simulink model "gm_uz_pmsm_model_6ph_dqxy_vnl"  (R2024b)
settings: Solver=FixedStepAuto  StartTime=0.0  StopTime=0.5  RelTol=1e-3
PreLoadFcn:
  | uz_pmsm_model_6ph_dqxy_init_parameter
undefined symbols (not defined in the file or in its folder): friction_coefficient, inertia, k_i_d, k_i_x, k_i_y, k_p_d, k_p_q, k_p_x, k_p_y, L_d, L_q, L_x, L_y, polepair, psi_pm, R_1, setpoint_step, simulate_mechanical, simulate_open_loop, static_friction_torque, ts
libraries: hdlmdlgenlib x5, slpidlib x4, simulink x2
(part 1 of 2)
settings Model: Creator=ts  LastModifiedBy=hufnagelde
settings SolverCC: AlgebraicLoopSolver=TrustRegion  AutoInsertRateTranBlk=on
settings DataIOCC: LimitDataPoints=on  SaveOutput=off  SaveTime=off
settings OptimizationCC: BlockReduction=off  ConditionallyExecuteInputs=off  DefaultParameterBehavior=Inlined  LifeSpan=inf
settings DebuggingCC: AlgebraicLoopMsg=error  InheritedTsInSrcMsg=none  SingleTaskRateTransMsg=error  UnconnectedInputMsg=warning  UnconnectedOutputMsg=warning  UnconnectedLineMsg=warning  AllowSymbolicDim=off  StrictBusMsg=ErrorOnBusTreatedAsVector  SFUnexpectedBacktrackingDiag=warning  SFNoUnconditionalDefaultTransitionDiag=warning  SFExecutionAtInitializationDiag=none  ArithmeticOperatorsInVariantConditions=warning
settings HardwareCC: ProdBitPerPointer=32  ProdBitPerSizeT=32  ProdBitPerPtrDiffT=32  ProdLargestAtomicFloat=None  ProdIntDivRoundTo=Undefined  ProdEndianess=Unspecified  ProdWordSize=32  ProdHWDeviceType=ASIC/FPGA->ASIC/FPGA  ProdEqTarget=off
settings ModelReferenceCC: EnableRefExpFcnMdlSchedulingChecks=on
settings SFSimCC: SimUseLocalCustomCode=off  CustomCodeUndefinedFunction=UseInterfaceOnly
settings RTWCC: RTWUseLocalCustomCode=off  GPUComputeCapability=3.5  DLArmComputeVersion=19.05
settings CodeAppCC: StateflowObjectComments=on
settings GRTTargetCC: TargetLangStandard=C89/C90 (ANSI)
settings ConfigComp: CovScope=ReferencedModels  CovMetricSettings=dw  CovSaveCumulativeToWorkspaceVar=on  CovSaveSingleToWorkspaceVar=on  CovExternalEMLEnable=off  CovSFcnEnable=off

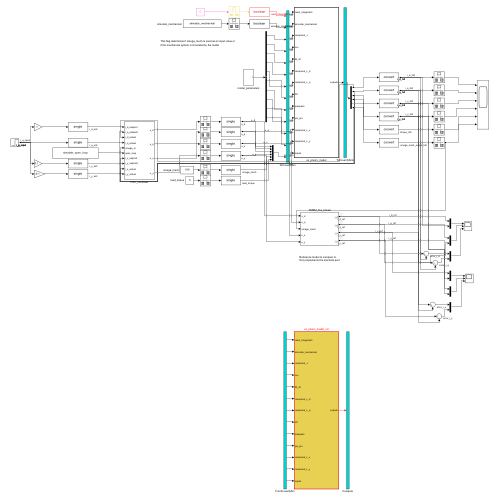
[thumbnail: Simulink's stored preview of the top-level diagram]
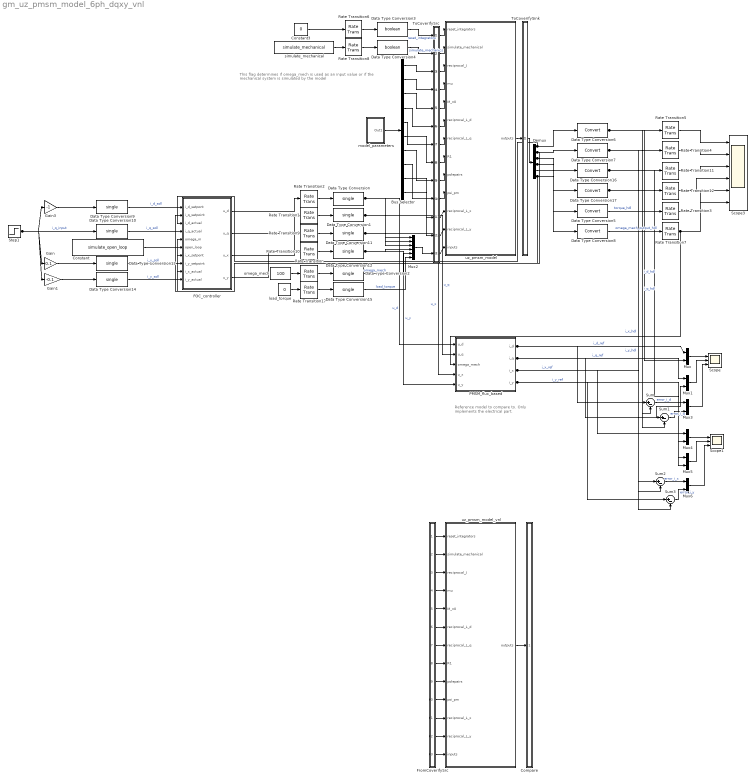
== system gm_uz_pmsm_model_6ph_dqxy_vnl ==
  note: Reference model to compare to.
      | Only implements the electrical part.
  note: This flag determines if omega_mech is used as an input value or
      | if the mechanical system is simulated by the model
  Bus Selector : BusSelector  OutputSignals=1_J,mu,M_R0,1_L_d,1_L_q,R_1,polepair,psi_pm,1_L_x,1_L_y
  Compare : Subsystem
      mask Display: disp('')
  Constant : Constant  Value=simulate_open_loop
  Constant3 : Constant  Value=0
  Data Type Conversion{,1..2,9..15} (10 alike) : DataTypeConversion  OutDataTypeStr=single  SaturateOnIntegerOverflow=off  RndMeth=Floor
  Data Type Conversion{5..8,16..17} (6 alike) : DataTypeConversion  SaturateOnIntegerOverflow=off  RndMeth=Floor
  Data Type Conversion3 : DataTypeConversion  OutDataTypeStr=boolean  SaturateOnIntegerOverflow=off  RndMeth=Floor
  Data Type Conversion4 : DataTypeConversion  OutDataTypeStr=boolean  SaturateOnIntegerOverflow=off  RndMeth=Floor
  Demux : Demux  Outputs=6
  FOC_controller : Subsystem
  FromCoverifySrc : Subsystem
      mask Display: disp('')
  Gain : Gain  Gain=0.1
  Gain1 : Gain  Gain=-0.1
  Gain3 : Gain  Gain=-1
  Mux{,1,3..6} (6 alike) : Mux  Inputs=2
  Mux2 : Mux  Inputs=6
  PMSM_flux_based : Subsystem
  Rate Transition{,1..2,6,8..10,17} (8 alike) : RateTransition  OutPortSampleTime=ts
  Rate Transition{3..5,7,11..12} (6 alike) : RateTransition
  Scope : Scope  NumInputPorts=3
  Scope1 : Scope  NumInputPorts=3
  Scope3 : Scope  NumInputPorts=6
  Step1 : Step  Time=0.2  After=setpoint_step
  Sum{,1..3} (4 alike) : Sum  Inputs=|+-
  ToCoverifySink : Subsystem
      mask Display: disp('')
  ToCoverifySrc : Subsystem
      mask Display: disp('')
  load_torque : Constant  Value=0
  model_parameters : Subsystem
  omega_mech : Constant  Value=100
  simulate_mechanical : Constant  Value=simulate_mechanical
  uz_pmsm_model : Subsystem  TreatAsAtomicUnit=on
  uz_pmsm_model_vnl : Subsystem  TreatAsAtomicUnit=on
  wires:
  Rate Transition/1 -> Data Type Conversion2/1
  Data Type Conversion6/1 -> Mux/2, Sum/2, Rate Transition5/1  "i_d_hdl"
  Data Type Conversion7/1 -> Mux1/2, Sum1/2, Rate Transition4/1  "i_q_hdl"
  Data Type Conversion5/1 -> Rate Transition3/1  "torque_hdl"
  Rate Transition4/1 -> Scope3/2
  Rate Transition5/1 -> Scope3/1
  Rate Transition3/1 -> Scope3/5
  Rate Transition6/1 -> Data Type Conversion3/1
  Constant3/1 -> Rate Transition6/1
  Rate Transition8/1 -> Data Type Conversion4/1
  simulate_mechanical/1 -> Rate Transition8/1
  load_torque/1 -> Rate Transition17/1
  Rate Transition17/1 -> Data Type Conversion15/1
  Mux/1 -> Scope/1
  Mux1/1 -> Scope/2
  PMSM_flux_based/2(i_q) -> Mux1/1, Sum1/1  "i_q_ref"
  PMSM_flux_based/1(i_d) -> Mux/1, Sum/1  "i_d_ref"
  Data Type Conversion8/1 -> Rate Transition7/1  "omega_mech_output_hdl"
  Rate Transition7/1 -> PMSM_flux_based/3(omega_mech), Scope3/6
  model_parameters/1(Out1) -> Bus Selector/1
  Sum/1 -> Mux3/1  "error_i_d"
  Sum1/1 -> Mux3/2  "error_i_q"
  Mux3/1 -> Scope/3
  Step1/1 -> Gain1/1, Gain/1, Gain3/1, Data Type Conversion10/1  "i_q_input"
  Demux/5 -> Data Type Conversion5/1
  Gain3/1 -> Data Type Conversion9/1
  Demux/1 -> FOC_controller/3(i_d_actual), Data Type Conversion6/1
  Demux/6 -> FOC_controller/5(omega_m), Data Type Conversion8/1
  Demux/2 -> FOC_controller/4(i_q_actual), Data Type Conversion7/1
  Data Type Conversion/1 -> PMSM_flux_based/1(u_d), Mux2/1  "u_d"
  Data Type Conversion1/1 -> PMSM_flux_based/2(u_q), Mux2/2  "u_q"
  Data Type Conversion15/1 -> Mux2/6  "load_torque"
  Data Type Conversion2/1 -> Mux2/5  "omega_mech"
  Data Type Conversion9/1 -> FOC_controller/1(i_d_setpont)  "i_d_soll"
  Data Type Conversion10/1 -> FOC_controller/2(i_q_setpoint)  "i_q_soll"
  omega_mech/1 -> Rate Transition/1
  Constant/1 -> FOC_controller/6(open_loop)
  Rate Transition9/1 -> Data Type Conversion11/1
  Rate Transition10/1 -> Data Type Conversion12/1
  Rate Transition1/1 -> Data Type Conversion1/1
  Rate Transition2/1 -> Data Type Conversion/1
  FOC_controller/1(u_d) -> Rate Transition2/1
  FOC_controller/2(u_q) -> Rate Transition1/1
  FOC_controller/3(u_x) -> Rate Transition9/1
  FOC_controller/4(u_y) -> Rate Transition10/1
  Data Type Conversion11/1 -> PMSM_flux_based/4(u_x), Mux2/3  "u_x"
  Data Type Conversion12/1 -> PMSM_flux_based/5(u_y), Mux2/4  "u_y"
  Gain1/1 -> Data Type Conversion14/1
  Gain/1 -> Data Type Conversion13/1
  Data Type Conversion13/1 -> FOC_controller/7(i_x_setpont)  "i_x_soll"
  Data Type Conversion14/1 -> FOC_controller/8(i_y_setpoint)  "i_y_soll"
  Data Type Conversion16/1 -> Sum2/2, Mux4/2, Rate Transition11/1  "i_x_hdl"
  Rate Transition11/1 -> Scope3/3
  Demux/3 -> FOC_controller/9(i_x_actual), Data Type Conversion16/1
  Data Type Conversion17/1 -> Sum3/2, Mux5/2, Rate Transition12/1  "i_y_hdl"
  Rate Transition12/1 -> Scope3/4
  Demux/4 -> FOC_controller/10(i_y_actual), Data Type Conversion17/1
  Mux4/1 -> Scope1/1
  PMSM_flux_based/3(i_x) -> Sum2/1, Mux4/1  "i_x_ref"
  PMSM_flux_based/4(i_y) -> Mux5/1, Sum3/1  "i_y_ref"
  Mux5/1 -> Scope1/2
  Sum2/1 -> Mux6/1  "error_i_x"
  Sum3/1 -> Mux6/2  "error_i_y"
  Mux6/1 -> Scope1/3
  ToCoverifySrc/1(out1) -> uz_pmsm_model/1(reset_integrators)
  ToCoverifySrc/2(out2) -> uz_pmsm_model/2(simulate_mechanical)
  ToCoverifySrc/3(out3) -> uz_pmsm_model/3(reciprocal_J)
  ToCoverifySrc/4(out4) -> uz_pmsm_model/4(mu)
  ToCoverifySrc/5(out5) -> uz_pmsm_model/5(M_n0)
  ToCoverifySrc/6(out6) -> uz_pmsm_model/6(reciprocal_L_d)
  ToCoverifySrc/7(out7) -> uz_pmsm_model/7(reciprocal_L_q)
  ToCoverifySrc/8(out8) -> uz_pmsm_model/8(R1)
  ToCoverifySrc/9(out9) -> uz_pmsm_model/9(polepairs)
  ToCoverifySrc/10(out10) -> uz_pmsm_model/10(psi_pm)
  ToCoverifySrc/11(out11) -> uz_pmsm_model/11(reciprocal_L_x)
  ToCoverifySrc/12(out12) -> uz_pmsm_model/12(reciprocal_L_y)
  ToCoverifySrc/13(out13) -> uz_pmsm_model/13(inputs)
  uz_pmsm_model/1(outputs) -> ToCoverifySink/1(in1)
  Data Type Conversion3/1 -> ToCoverifySrc/1(in1)  "reset_integrators"
  Data Type Conversion4/1 -> ToCoverifySrc/2(in2)  "simulate_mechanics"
  Bus Selector/1 -> ToCoverifySrc/3(in3)
  Bus Selector/2 -> ToCoverifySrc/4(in4)
  Bus Selector/3 -> ToCoverifySrc/5(in5)
  Bus Selector/4 -> ToCoverifySrc/6(in6)
  Bus Selector/5 -> ToCoverifySrc/7(in7)
  Bus Selector/6 -> ToCoverifySrc/8(in8)
  Bus Selector/7 -> ToCoverifySrc/9(in9)
  Bus Selector/8 -> ToCoverifySrc/10(in10)
  Bus Selector/9 -> ToCoverifySrc/11(in11)
  Bus Selector/10 -> ToCoverifySrc/12(in12)
  Mux2/1 -> ToCoverifySrc/13(in13)
  ToCoverifySink/1(out1) -> Demux/1
  FromCoverifySrc/1(out1) -> uz_pmsm_model_vnl/1(reset_integrators)
  FromCoverifySrc/2(out2) -> uz_pmsm_model_vnl/2(simulate_mechanical)
  FromCoverifySrc/3(out3) -> uz_pmsm_model_vnl/3(reciprocal_J)
  FromCoverifySrc/4(out4) -> uz_pmsm_model_vnl/4(mu)
  FromCoverifySrc/5(out5) -> uz_pmsm_model_vnl/5(M_n0)
  FromCoverifySrc/6(out6) -> uz_pmsm_model_vnl/6(reciprocal_L_d)
  FromCoverifySrc/7(out7) -> uz_pmsm_model_vnl/7(reciprocal_L_q)
  FromCoverifySrc/8(out8) -> uz_pmsm_model_vnl/8(R1)
  FromCoverifySrc/9(out9) -> uz_pmsm_model_vnl/9(polepairs)
  FromCoverifySrc/10(out10) -> uz_pmsm_model_vnl/10(psi_pm)
  FromCoverifySrc/11(out11) -> uz_pmsm_model_vnl/11(reciprocal_L_x)
  FromCoverifySrc/12(out12) -> uz_pmsm_model_vnl/12(reciprocal_L_y)
  FromCoverifySrc/13(out13) -> uz_pmsm_model_vnl/13(inputs)
  uz_pmsm_model_vnl/1(outputs) -> Compare/1(in1)

== system gm_uz_pmsm_model_6ph_dqxy_vnl/Compare ==
  in1 : Inport
  Assert_outputs : Subsystem  mask{ToleranceValue=1e-07}
  CleanupScopes : Subsystem
      settings: OpenFcn=|
      | blkName = gcb; %self block
      | idx = regexp(blkName, '/CleanupScopes$', 'once');
      | blkParent = blkName(1:idx-1);
      | blks=find_system(blkParent, 'LookUnderMasks', 'all','blocktype', 'Scope');
      | for itr = 1:length(blks)
      | 	 hScopeCfg = get_param(blks{itr},'ScopeConfiguration');
      | 	 hScopeCfg.Visible = ~ hScopeCfg.Visible;
      | end
      | drawnow;
      mask Display: fprintf(message('hdlcoder:cosim:vnl_dblclick').getString());
  Enable : Subsystem
      settings: OpenFcn=|
      | blkName = gcb;
      | idx = regexp(blkName, '/Enable$', 'once');
      | blkParent = blkName(1:idx-1);
      | blks=find_system(blkParent, 'LookUnderMasks', 'all','blocktype', 'Assertion');
      | e = get_param(blks{1}, 'Enabled');
      | if strcmp(e, 'on'), f= 'off';, else, f = 'on';, end
      | for ii=1:length(blks), set_param(blks{ii}, 'Enabled', f);, end
      | set_param(gcb, 'MaskDisplay',['fprintf(message(''hdlcoder:cosim:vnl_dblclick_assertions'',','''',upper(e),'''',').getString())']);
      mask Display: fprintf(message('hdlcoder:cosim:vnl_dblclick_assertions','OFF').getString());
  pathdelay1 : Delay  DelayLength=1
  wires:
  in1/1 -> pathdelay1/1
  pathdelay1/1 -> Assert_outputs/1(cosim)
  [out1] -> Assert_outputs/2(dut)

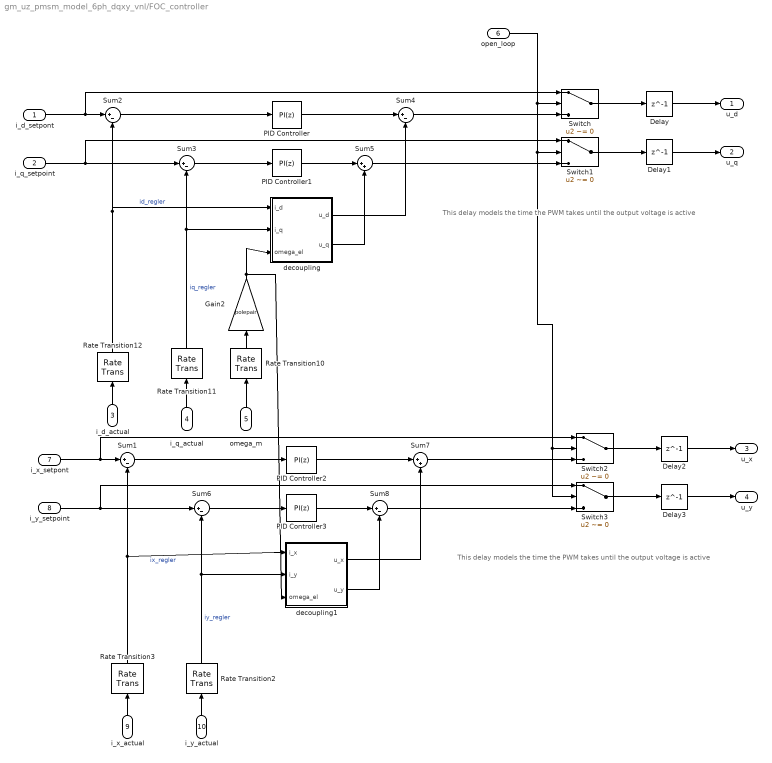
== system gm_uz_pmsm_model_6ph_dqxy_vnl/FOC_controller ==
  note: This delay models the time the PWM takes until the output voltage is active
  note: This delay models the time the PWM takes until the output voltage is active
  i_d_setpont : Inport
  i_q_setpoint : Inport  Port=2
  i_d_actual : Inport  Port=3
  i_q_actual : Inport  Port=4
  omega_m : Inport  Port=5
  open_loop : Inport  Port=6
  i_x_setpont : Inport  Port=7
  i_y_setpoint : Inport  Port=8
  i_x_actual : Inport  Port=9
  i_y_actual : Inport  Port=10
  Delay{,1..3} (4 alike) : Delay  DelayLength=1
  Gain2 : Gain  Gain=polepair
  PID Controller : slpidlib/PID Controller  Controller=PI  Form=Parallel  TimeDomain=Discrete-time  UseExternalTs=off  SampleTime=-1  IntegratorMethod=Forward Euler  FilterMethod=Forward Euler  ControllerParametersSource=internal  P=k_p_d  I=k_i_d  UseKiTs=off  D=0  UseExternalDerivativeSource=off  N=100  UseFilter=on  TunerSelectOption=Transfer Function Based (PID Tuner App)  InitialConditionSource=internal  InitialConditionForIntegrator=0  InitialConditionForFilter=0  DifferentiatorICPrevScaledInput=0  ExternalReset=none  TrackingMode=off  Kt=1  LimitOutput=off  SatLimitsSource=internal  UpperSaturationLimit=inf  LowerSaturationLimit=-inf  LinearizeAsGain=on  AntiWindupMode=none  Kb=1  LimitIntegrator=off  UpperIntegratorSaturationLimit=inf  LowerIntegratorSaturationLimit=-inf  POutMin=[]  POutMax=[]  IOutMin=[]  IOutMax=[]  DOutMin=[]  DOutMax=[]  NOutMin=[]  NOutMax=[]  SumOutMin=[]  SumOutMax=[]  SaturationOutMin=[]  SaturationOutMax=[]  PParamMin=[]  PParamMax=[]  IParamMin=[]  IParamMax=[]  DParamMin=[]  DParamMax=[]  NParamMin=[]  NParamMax=[]  KbParamMin=[]  KbParamMax=[]  KtParamMin=[]  KtParamMax=[]  KbOutMin=[]  KbOutMax=[]  KtOutMin=[]  KtOutMax=[]  IntegratorOutMin=[]  IntegratorOutMax=[]  FilterOutMin=[]  FilterOutMax=[]  SumI1OutMin=[]  SumI1OutMax=[]  SumI2OutMin=[]  SumI2OutMax=[]  SumI3OutMin=[]  SumI3OutMax=[]  SumI4OutMin=[]  SumI4OutMax=[]  SumDOutMin=[]  SumDOutMax=[]  DifferentiatorOutMin=[]  DifferentiatorOutMax=[]  FilterDiffOutCoefMin=[]  FilterDiffOutCoefMax=[]  ReciprocalOutMin=[]  ReciprocalOutMax=[]  SumDenOutMin=[]  SumDenOutMax=[]  SumNumOutMin=[]  SumNumOutMax=[]  DivideOutMin=[]  DivideOutMax=[]  UdiffTsProdOutMin=[]  UdiffTsProdOutMax=[]  NTsProdOutMin=[]  NTsProdOutMax=[]  UintegralTsProdOutMin=[]  UintegralTsProdOutMax=[]  UngainTsProdOutMin=[]  UngainTsProdOutMax=[]  ClampingZeroOutDataTypeStr=Inherit: Inherit via back propagation  ClampingZeroOutMin=[]  ClampingZeroOutMax=[]  FilterDenConstantOutDataTypeStr=Inherit: Inherit via back propagation  FilterDenConstantOutMin=[]  FilterDenConstantOutMax=[]  PCopyOutDataTypeStr=Inherit: Inherit via back propagation  PCopyOutMin=[]  PCopyOutMax=[]  NCopyOutDataTypeStr=Inherit: Inherit via back propagation  NCopyOutMin=[]  NCopyOutMax=[]  IntegratorContinuousStateAttributes=''  IntegratorStateMustResolveToSignalObject=off  IntegratorRTWStateStorageClass=Auto  FilterContinuousStateAttributes=''  FilterStateMustResolveToSignalObject=off  FilterRTWStateStorageClass=Auto  ParallelPVariant=InternalParameters  IdealPVariant=Disabled  IVariant=InternalParameters  DVariant=Disabled  IntegratorVariant=Discrete  SatVariant=Disabled  AWVariant=Passthrough  PCopyVariant=Disabled  TRVariant=Disabled  FdbkBlocksVariant=Forward  IdealPFdbkVariant=Disabled  SatFdbkVariant=Disabled  DerivativeFilterVariant=Disabled  NVariant=Disabled  NCopyVariant=Disabled_SignalSpec  FilterICVariant=Disabled  IntegratorICVariant=InternalICs  ExternalResetVariant=Disabled  TRSumVariant=Passthrough  SumFdbkVariant=Disabled  SumVariant=Sum_PI  TsampFilterVariant=InternalTs  TsampNgainVariant=Passthrough  TsampIntegralVariant=Disabled_SignalSpec  ExternalSaturationOutDataTypeStr=Inherit: Same as second input  DerivativeSourceVariant=Disabled  PreIntVariant=InternalPreInt
  PID Controller1 : slpidlib/PID Controller  Controller=PI  Form=Parallel  TimeDomain=Discrete-time  UseExternalTs=off  SampleTime=-1  IntegratorMethod=Forward Euler  FilterMethod=Forward Euler  ControllerParametersSource=internal  P=k_p_q  I=k_i_d  UseKiTs=off  D=0  UseExternalDerivativeSource=off  N=100  UseFilter=on  TunerSelectOption=Transfer Function Based (PID Tuner App)  InitialConditionSource=internal  InitialConditionForIntegrator=0  InitialConditionForFilter=0  DifferentiatorICPrevScaledInput=0  ExternalReset=none  TrackingMode=off  Kt=1  LimitOutput=off  SatLimitsSource=internal  UpperSaturationLimit=inf  LowerSaturationLimit=-inf  LinearizeAsGain=on  AntiWindupMode=none  Kb=1  LimitIntegrator=off  UpperIntegratorSaturationLimit=inf  LowerIntegratorSaturationLimit=-inf  POutMin=[]  POutMax=[]  IOutMin=[]  IOutMax=[]  DOutMin=[]  DOutMax=[]  NOutMin=[]  NOutMax=[]  SumOutMin=[]  SumOutMax=[]  SaturationOutMin=[]  SaturationOutMax=[]  PParamMin=[]  PParamMax=[]  IParamMin=[]  IParamMax=[]  DParamMin=[]  DParamMax=[]  NParamMin=[]  NParamMax=[]  KbParamMin=[]  KbParamMax=[]  KtParamMin=[]  KtParamMax=[]  KbOutMin=[]  KbOutMax=[]  KtOutMin=[]  KtOutMax=[]  IntegratorOutMin=[]  IntegratorOutMax=[]  FilterOutMin=[]  FilterOutMax=[]  SumI1OutMin=[]  SumI1OutMax=[]  SumI2OutMin=[]  SumI2OutMax=[]  SumI3OutMin=[]  SumI3OutMax=[]  SumI4OutMin=[]  SumI4OutMax=[]  SumDOutMin=[]  SumDOutMax=[]  DifferentiatorOutMin=[]  DifferentiatorOutMax=[]  FilterDiffOutCoefMin=[]  FilterDiffOutCoefMax=[]  ReciprocalOutMin=[]  ReciprocalOutMax=[]  SumDenOutMin=[]  SumDenOutMax=[]  SumNumOutMin=[]  SumNumOutMax=[]  DivideOutMin=[]  DivideOutMax=[]  UdiffTsProdOutMin=[]  UdiffTsProdOutMax=[]  NTsProdOutMin=[]  NTsProdOutMax=[]  UintegralTsProdOutMin=[]  UintegralTsProdOutMax=[]  UngainTsProdOutMin=[]  UngainTsProdOutMax=[]  ClampingZeroOutDataTypeStr=Inherit: Inherit via back propagation  ClampingZeroOutMin=[]  ClampingZeroOutMax=[]  FilterDenConstantOutDataTypeStr=Inherit: Inherit via back propagation  FilterDenConstantOutMin=[]  FilterDenConstantOutMax=[]  PCopyOutDataTypeStr=Inherit: Inherit via back propagation  PCopyOutMin=[]  PCopyOutMax=[]  NCopyOutDataTypeStr=Inherit: Inherit via back propagation  NCopyOutMin=[]  NCopyOutMax=[]  IntegratorContinuousStateAttributes=''  IntegratorStateMustResolveToSignalObject=off  IntegratorRTWStateStorageClass=Auto  FilterContinuousStateAttributes=''  FilterStateMustResolveToSignalObject=off  FilterRTWStateStorageClass=Auto  ParallelPVariant=InternalParameters  IdealPVariant=Disabled  IVariant=InternalParameters  DVariant=Disabled  IntegratorVariant=Discrete  SatVariant=Disabled  AWVariant=Passthrough  PCopyVariant=Disabled  TRVariant=Disabled  FdbkBlocksVariant=Forward  IdealPFdbkVariant=Disabled  SatFdbkVariant=Disabled  DerivativeFilterVariant=Disabled  NVariant=Disabled  NCopyVariant=Disabled_SignalSpec  FilterICVariant=Disabled  IntegratorICVariant=InternalICs  ExternalResetVariant=Disabled  TRSumVariant=Passthrough  SumFdbkVariant=Disabled  SumVariant=Sum_PI  TsampFilterVariant=InternalTs  TsampNgainVariant=Passthrough  TsampIntegralVariant=Disabled_SignalSpec  ExternalSaturationOutDataTypeStr=Inherit: Same as second input  DerivativeSourceVariant=Disabled  PreIntVariant=InternalPreInt
  PID Controller2 : slpidlib/PID Controller  Controller=PI  Form=Parallel  TimeDomain=Discrete-time  UseExternalTs=off  SampleTime=-1  IntegratorMethod=Forward Euler  FilterMethod=Forward Euler  ControllerParametersSource=internal  P=k_p_x  I=k_i_x  UseKiTs=off  D=0  UseExternalDerivativeSource=off  N=100  UseFilter=on  TunerSelectOption=Transfer Function Based (PID Tuner App)  InitialConditionSource=internal  InitialConditionForIntegrator=0  InitialConditionForFilter=0  DifferentiatorICPrevScaledInput=0  ExternalReset=none  TrackingMode=off  Kt=1  LimitOutput=off  SatLimitsSource=internal  UpperSaturationLimit=inf  LowerSaturationLimit=-inf  LinearizeAsGain=on  AntiWindupMode=none  Kb=1  LimitIntegrator=off  UpperIntegratorSaturationLimit=inf  LowerIntegratorSaturationLimit=-inf  POutMin=[]  POutMax=[]  IOutMin=[]  IOutMax=[]  DOutMin=[]  DOutMax=[]  NOutMin=[]  NOutMax=[]  SumOutMin=[]  SumOutMax=[]  SaturationOutMin=[]  SaturationOutMax=[]  PParamMin=[]  PParamMax=[]  IParamMin=[]  IParamMax=[]  DParamMin=[]  DParamMax=[]  NParamMin=[]  NParamMax=[]  KbParamMin=[]  KbParamMax=[]  KtParamMin=[]  KtParamMax=[]  KbOutMin=[]  KbOutMax=[]  KtOutMin=[]  KtOutMax=[]  IntegratorOutMin=[]  IntegratorOutMax=[]  FilterOutMin=[]  FilterOutMax=[]  SumI1OutMin=[]  SumI1OutMax=[]  SumI2OutMin=[]  SumI2OutMax=[]  SumI3OutMin=[]  SumI3OutMax=[]  SumI4OutMin=[]  SumI4OutMax=[]  SumDOutMin=[]  SumDOutMax=[]  DifferentiatorOutMin=[]  DifferentiatorOutMax=[]  FilterDiffOutCoefMin=[]  FilterDiffOutCoefMax=[]  ReciprocalOutMin=[]  ReciprocalOutMax=[]  SumDenOutMin=[]  SumDenOutMax=[]  SumNumOutMin=[]  SumNumOutMax=[]  DivideOutMin=[]  DivideOutMax=[]  UdiffTsProdOutMin=[]  UdiffTsProdOutMax=[]  NTsProdOutMin=[]  NTsProdOutMax=[]  UintegralTsProdOutMin=[]  UintegralTsProdOutMax=[]  UngainTsProdOutMin=[]  UngainTsProdOutMax=[]  ClampingZeroOutDataTypeStr=Inherit: Inherit via back propagation  ClampingZeroOutMin=[]  ClampingZeroOutMax=[]  FilterDenConstantOutDataTypeStr=Inherit: Inherit via back propagation  FilterDenConstantOutMin=[]  FilterDenConstantOutMax=[]  PCopyOutDataTypeStr=Inherit: Inherit via back propagation  PCopyOutMin=[]  PCopyOutMax=[]  NCopyOutDataTypeStr=Inherit: Inherit via back propagation  NCopyOutMin=[]  NCopyOutMax=[]  IntegratorContinuousStateAttributes=''  IntegratorStateMustResolveToSignalObject=off  IntegratorRTWStateStorageClass=Auto  FilterContinuousStateAttributes=''  FilterStateMustResolveToSignalObject=off  FilterRTWStateStorageClass=Auto  ParallelPVariant=InternalParameters  IdealPVariant=Disabled  IVariant=InternalParameters  DVariant=Disabled  IntegratorVariant=Discrete  SatVariant=Disabled  AWVariant=Passthrough  PCopyVariant=Disabled  TRVariant=Disabled  FdbkBlocksVariant=Forward  IdealPFdbkVariant=Disabled  SatFdbkVariant=Disabled  DerivativeFilterVariant=Disabled  NVariant=Disabled  NCopyVariant=Disabled_SignalSpec  FilterICVariant=Disabled  IntegratorICVariant=InternalICs  ExternalResetVariant=Disabled  TRSumVariant=Passthrough  SumFdbkVariant=Disabled  SumVariant=Sum_PI  TsampFilterVariant=InternalTs  TsampNgainVariant=Passthrough  TsampIntegralVariant=Disabled_SignalSpec  ExternalSaturationOutDataTypeStr=Inherit: Same as second input  DerivativeSourceVariant=Disabled  PreIntVariant=InternalPreInt
  PID Controller3 : slpidlib/PID Controller  Controller=PI  Form=Parallel  TimeDomain=Discrete-time  UseExternalTs=off  SampleTime=-1  IntegratorMethod=Forward Euler  FilterMethod=Forward Euler  ControllerParametersSource=internal  P=k_p_y  I=k_i_y  UseKiTs=off  D=0  UseExternalDerivativeSource=off  N=100  UseFilter=on  TunerSelectOption=Transfer Function Based (PID Tuner App)  InitialConditionSource=internal  InitialConditionForIntegrator=0  InitialConditionForFilter=0  DifferentiatorICPrevScaledInput=0  ExternalReset=none  TrackingMode=off  Kt=1  LimitOutput=off  SatLimitsSource=internal  UpperSaturationLimit=inf  LowerSaturationLimit=-inf  LinearizeAsGain=on  AntiWindupMode=none  Kb=1  LimitIntegrator=off  UpperIntegratorSaturationLimit=inf  LowerIntegratorSaturationLimit=-inf  POutMin=[]  POutMax=[]  IOutMin=[]  IOutMax=[]  DOutMin=[]  DOutMax=[]  NOutMin=[]  NOutMax=[]  SumOutMin=[]  SumOutMax=[]  SaturationOutMin=[]  SaturationOutMax=[]  PParamMin=[]  PParamMax=[]  IParamMin=[]  IParamMax=[]  DParamMin=[]  DParamMax=[]  NParamMin=[]  NParamMax=[]  KbParamMin=[]  KbParamMax=[]  KtParamMin=[]  KtParamMax=[]  KbOutMin=[]  KbOutMax=[]  KtOutMin=[]  KtOutMax=[]  IntegratorOutMin=[]  IntegratorOutMax=[]  FilterOutMin=[]  FilterOutMax=[]  SumI1OutMin=[]  SumI1OutMax=[]  SumI2OutMin=[]  SumI2OutMax=[]  SumI3OutMin=[]  SumI3OutMax=[]  SumI4OutMin=[]  SumI4OutMax=[]  SumDOutMin=[]  SumDOutMax=[]  DifferentiatorOutMin=[]  DifferentiatorOutMax=[]  FilterDiffOutCoefMin=[]  FilterDiffOutCoefMax=[]  ReciprocalOutMin=[]  ReciprocalOutMax=[]  SumDenOutMin=[]  SumDenOutMax=[]  SumNumOutMin=[]  SumNumOutMax=[]  DivideOutMin=[]  DivideOutMax=[]  UdiffTsProdOutMin=[]  UdiffTsProdOutMax=[]  NTsProdOutMin=[]  NTsProdOutMax=[]  UintegralTsProdOutMin=[]  UintegralTsProdOutMax=[]  UngainTsProdOutMin=[]  UngainTsProdOutMax=[]  ClampingZeroOutDataTypeStr=Inherit: Inherit via back propagation  ClampingZeroOutMin=[]  ClampingZeroOutMax=[]  FilterDenConstantOutDataTypeStr=Inherit: Inherit via back propagation  FilterDenConstantOutMin=[]  FilterDenConstantOutMax=[]  PCopyOutDataTypeStr=Inherit: Inherit via back propagation  PCopyOutMin=[]  PCopyOutMax=[]  NCopyOutDataTypeStr=Inherit: Inherit via back propagation  NCopyOutMin=[]  NCopyOutMax=[]  IntegratorContinuousStateAttributes=''  IntegratorStateMustResolveToSignalObject=off  IntegratorRTWStateStorageClass=Auto  FilterContinuousStateAttributes=''  FilterStateMustResolveToSignalObject=off  FilterRTWStateStorageClass=Auto  ParallelPVariant=InternalParameters  IdealPVariant=Disabled  IVariant=InternalParameters  DVariant=Disabled  IntegratorVariant=Discrete  SatVariant=Disabled  AWVariant=Passthrough  PCopyVariant=Disabled  TRVariant=Disabled  FdbkBlocksVariant=Forward  IdealPFdbkVariant=Disabled  SatFdbkVariant=Disabled  DerivativeFilterVariant=Disabled  NVariant=Disabled  NCopyVariant=Disabled_SignalSpec  FilterICVariant=Disabled  IntegratorICVariant=InternalICs  ExternalResetVariant=Disabled  TRSumVariant=Passthrough  SumFdbkVariant=Disabled  SumVariant=Sum_PI  TsampFilterVariant=InternalTs  TsampNgainVariant=Passthrough  TsampIntegralVariant=Disabled_SignalSpec  ExternalSaturationOutDataTypeStr=Inherit: Same as second input  DerivativeSourceVariant=Disabled  PreIntVariant=InternalPreInt
  Rate Transition{2..3,10..12} (5 alike) : RateTransition  OutPortSampleTime=ts_regler
  Sum{1..4,6,8} (6 alike) : Sum  Inputs=|+-
  Sum5 : Sum  Inputs=|++
  Sum7 : Sum  Inputs=|++
  Switch{,1..3} (4 alike) : Switch  Criteria=u2 ~= 0  SaturateOnIntegerOverflow=off  InputSameDT=off
  decoupling : Subsystem
  decoupling1 : Subsystem
  u_d : Outport
  u_q : Outport  Port=2
  u_x : Outport  Port=3
  u_y : Outport  Port=4
  wires:
  PID Controller/1 -> Sum4/1
  PID Controller1/1 -> Sum5/1
  Sum4/1 -> Switch/3
  i_d_actual/1 -> Rate Transition12/1
  i_d_setpont/1 -> Switch/1, Sum2/1
  Sum2/1 -> PID Controller/1
  Sum5/1 -> Switch1/3
  Sum3/1 -> PID Controller1/1
  i_q_actual/1 -> Rate Transition11/1
  Rate Transition12/1 -> decoupling/1(i_d), Sum2/2  "id_regler"
  Rate Transition11/1 -> decoupling/2(i_q), Sum3/2  "iq_regler"
  i_q_setpoint/1 -> Switch1/1, Sum3/1
  Rate Transition10/1 -> Gain2/1
  decoupling/1(u_d) -> Sum4/2
  decoupling/2(u_q) -> Sum5/2
  Switch/1 -> Delay/1
  Switch1/1 -> Delay1/1
  Delay/1 -> u_d/1
  Delay1/1 -> u_q/1
  Switch2/1 -> Delay2/1
  PID Controller3/1 -> Sum8/1
  Sum1/1 -> PID Controller2/1
  omega_m/1 -> Rate Transition10/1
  Delay2/1 -> u_x/1
  PID Controller2/1 -> Sum7/1
  Delay3/1 -> u_y/1
  Sum8/1 -> Switch3/3
  Sum6/1 -> PID Controller3/1
  Sum7/1 -> Switch2/3
  i_x_actual/1 -> Rate Transition3/1
  open_loop/1 -> Switch3/2, Switch2/2, Switch1/2, Switch/2
  i_y_setpoint/1 -> Switch3/1, Sum6/1
  i_y_actual/1 -> Rate Transition2/1
  Rate Transition2/1 -> decoupling1/2(i_y), Sum6/2  "iy_regler"
  decoupling1/2(u_y) -> Sum8/2
  i_x_setpont/1 -> Switch2/1, Sum1/1
  Switch3/1 -> Delay3/1
  Rate Transition3/1 -> decoupling1/1(i_x), Sum1/2  "ix_regler"
  decoupling1/1(u_x) -> Sum7/2
  Gain2/1 -> decoupling1/3(omega_el), decoupling/3(omega_el)

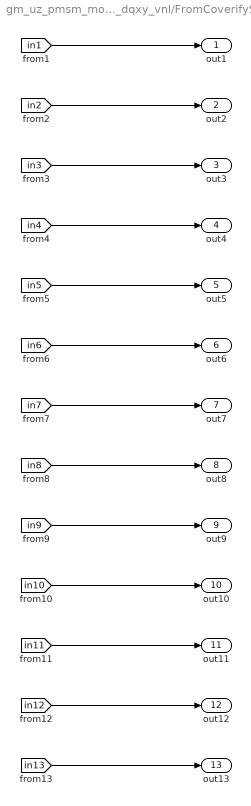
== system gm_uz_pmsm_model_6ph_dqxy_vnl/FromCoverifySrc ==
  out1 : Outport
  out2 : Outport  Port=2
  out3 : Outport  Port=3
  out4 : Outport  Port=4
  out5 : Outport  Port=5
  out6 : Outport  Port=6
  out7 : Outport  Port=7
  out8 : Outport  Port=8
  out9 : Outport  Port=9
  out10 : Outport  Port=10
  out11 : Outport  Port=11
  out12 : Outport  Port=12
  out13 : Outport  Port=13
  wires:
  [in1] -> out1/1
  [in2] -> out2/1
  [in3] -> out3/1
  [in4] -> out4/1
  [in5] -> out5/1
  [in6] -> out6/1
  [in7] -> out7/1
  [in8] -> out8/1
  [in9] -> out9/1
  [in10] -> out10/1
  [in11] -> out11/1
  [in12] -> out12/1
  [in13] -> out13/1

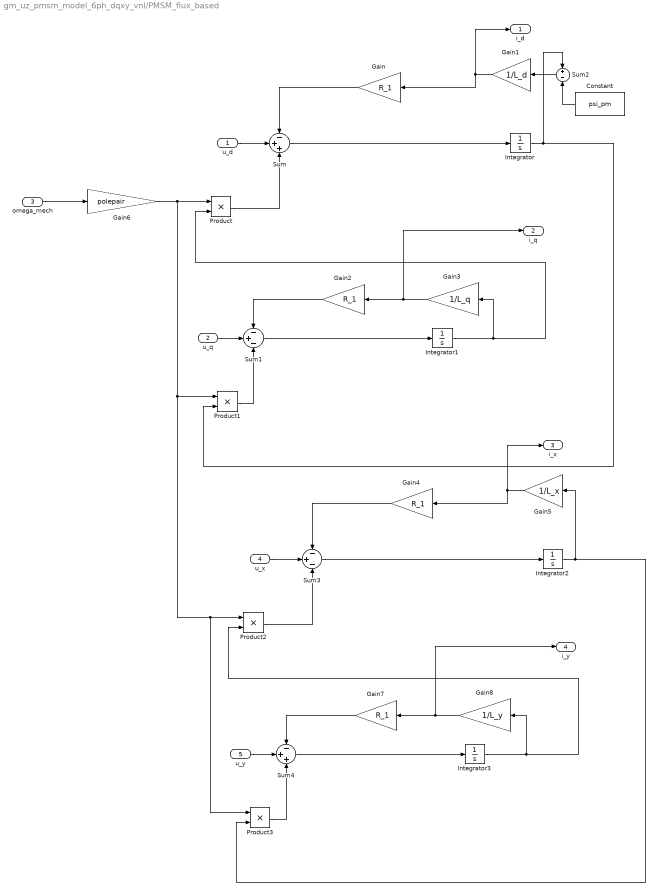
== system gm_uz_pmsm_model_6ph_dqxy_vnl/PMSM_flux_based ==
  u_d : Inport
  u_q : Inport  Port=2
  omega_mech : Inport  Port=3
  u_x : Inport  Port=4
  u_y : Inport  Port=5
  Constant : Constant  Value=psi_pm
  Gain{,2,4,7} (4 alike) : Gain  Gain=R_1
  Gain1 : Gain  Gain=1/L_d
  Gain3 : Gain  Gain=1/L_q
  Gain5 : Gain  Gain=1/L_x
  Gain6 : Gain  Gain=polepair
  Gain8 : Gain  Gain=1/L_y
  Integrator{,1..3} (4 alike) : Integrator
  Product{,1..3} (4 alike) : Product
  Sum : Sum  Inputs=-++
  Sum1 : Sum  Inputs=-+-
  Sum2 : Sum  Inputs=+-
  Sum3 : Sum  Inputs=-+-
  Sum4 : Sum  Inputs=-++
  i_d : Outport
  i_q : Outport  Port=2
  i_x : Outport  Port=3
  i_y : Outport  Port=4
  wires:
  u_d/1 -> Sum/2
  u_q/1 -> Sum1/2
  Sum/1 -> Integrator/1
  Gain/1 -> Sum/1
  Integrator/1 -> Product1/2, Sum2/1
  Constant/1 -> Sum2/2
  Sum2/1 -> Gain1/1
  Gain1/1 -> Gain/1, i_d/1
  Product/1 -> Sum/3
  Integrator1/1 -> Gain3/1, Product/2
  Product1/1 -> Sum1/3
  Sum1/1 -> Integrator1/1
  Gain2/1 -> Sum1/1
  Gain3/1 -> i_q/1, Gain2/1
  omega_mech/1 -> Gain6/1
  Gain5/1 -> Gain4/1, i_x/1
  Sum4/1 -> Integrator3/1
  Product3/1 -> Sum4/3
  Gain8/1 -> i_y/1, Gain7/1
  Gain6/1 -> Product3/1, Product2/1, Product1/1, Product/1
  Sum3/1 -> Integrator2/1
  Product2/1 -> Sum3/3
  Gain4/1 -> Sum3/1
  Integrator3/1 -> Gain8/1, Product2/2
  u_x/1 -> Sum3/2
  u_y/1 -> Sum4/2
  Gain7/1 -> Sum4/1
  Integrator2/1 -> Gain5/1, Product3/2

== system gm_uz_pmsm_model_6ph_dqxy_vnl/ToCoverifySink ==
  in1 : Inport
  out1 : Outport
  tag scope: out1=global
  wires:
  in1/1 -> out1/1, [out1]

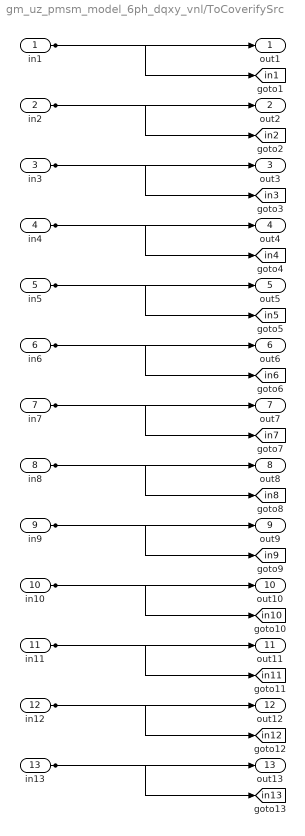
== system gm_uz_pmsm_model_6ph_dqxy_vnl/ToCoverifySrc ==
  in1 : Inport
  in2 : Inport  Port=2
  in3 : Inport  Port=3
  in4 : Inport  Port=4
  in5 : Inport  Port=5
  in6 : Inport  Port=6
  in7 : Inport  Port=7
  in8 : Inport  Port=8
  in9 : Inport  Port=9
  in10 : Inport  Port=10
  in11 : Inport  Port=11
  in12 : Inport  Port=12
  in13 : Inport  Port=13
  out1 : Outport
  out2 : Outport  Port=2
  out3 : Outport  Port=3
  out4 : Outport  Port=4
  out5 : Outport  Port=5
  out6 : Outport  Port=6
  out7 : Outport  Port=7
  out8 : Outport  Port=8
  out9 : Outport  Port=9
  out10 : Outport  Port=10
  out11 : Outport  Port=11
  out12 : Outport  Port=12
  out13 : Outport  Port=13
  tag scope: in10=global, in11=global, in12=global, in13=global, in1=global, in2=global, in3=global, in4=global, in5=global, in6=global, in7=global, in8=global, in9=global
  wires:
  in1/1 -> out1/1, [in1]
  in2/1 -> out2/1, [in2]
  in3/1 -> out3/1, [in3]
  in4/1 -> out4/1, [in4]
  in5/1 -> out5/1, [in5]
  in6/1 -> out6/1, [in6]
  in7/1 -> out7/1, [in7]
  in8/1 -> out8/1, [in8]
  in9/1 -> out9/1, [in9]
  in10/1 -> out10/1, [in10]
  in11/1 -> out11/1, [in11]
  in12/1 -> out12/1, [in12]
  in13/1 -> out13/1, [in13]

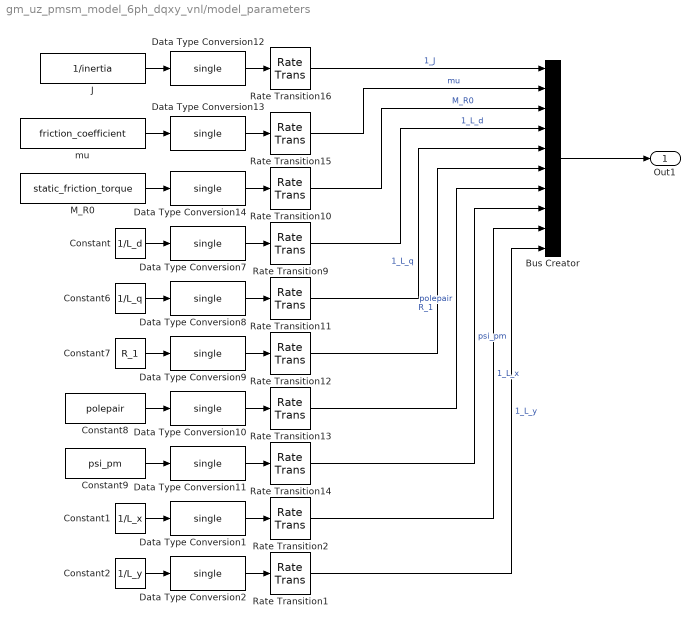
== system gm_uz_pmsm_model_6ph_dqxy_vnl/model_parameters ==
  Bus Creator : BusCreator  Inputs=10
  Constant : Constant  Value=1/L_d
  Constant1 : Constant  Value=1/L_x
  Constant2 : Constant  Value=1/L_y
  Constant6 : Constant  Value=1/L_q
  Constant7 : Constant  Value=R_1
  Constant8 : Constant  Value=polepair
  Constant9 : Constant  Value=psi_pm
  Data Type Conversion{1..2,7..14} (10 alike) : DataTypeConversion  OutDataTypeStr=single  SaturateOnIntegerOverflow=off  RndMeth=Floor
  J : Constant  Value=1/inertia
  M_R0 : Constant  Value=static_friction_torque
  Rate Transition{1..2,9..16} (10 alike) : RateTransition  OutPortSampleTime=ts
  mu : Constant  Value=friction_coefficient
  Out1 : Outport
  wires:
  Data Type Conversion12/1 -> Rate Transition16/1
  Data Type Conversion7/1 -> Rate Transition9/1
  Rate Transition10/1 -> Bus Creator/3  "M_R0"
  Rate Transition14/1 -> Bus Creator/8  "psi_pm"
  Data Type Conversion14/1 -> Rate Transition10/1
  Rate Transition12/1 -> Bus Creator/6  "R_1"
  Rate Transition16/1 -> Bus Creator/1  "1_J"
  Rate Transition13/1 -> Bus Creator/7  "polepair"
  Bus Creator/1 -> Out1/1
  Data Type Conversion11/1 -> Rate Transition14/1
  Constant8/1 -> Data Type Conversion10/1
  Data Type Conversion9/1 -> Rate Transition12/1
  Rate Transition15/1 -> Bus Creator/2  "mu"
  Constant6/1 -> Data Type Conversion8/1
  Rate Transition9/1 -> Bus Creator/4  "1_L_d"
  J/1 -> Data Type Conversion12/1
  Data Type Conversion8/1 -> Rate Transition11/1
  Data Type Conversion10/1 -> Rate Transition13/1
  mu/1 -> Data Type Conversion13/1
  M_R0/1 -> Data Type Conversion14/1
  Rate Transition11/1 -> Bus Creator/5  "1_L_q"
  Data Type Conversion13/1 -> Rate Transition15/1
  Constant7/1 -> Data Type Conversion9/1
  Constant9/1 -> Data Type Conversion11/1
  Constant/1 -> Data Type Conversion7/1
  Constant1/1 -> Data Type Conversion1/1
  Constant2/1 -> Data Type Conversion2/1
  Data Type Conversion1/1 -> Rate Transition2/1
  Data Type Conversion2/1 -> Rate Transition1/1
  Rate Transition2/1 -> Bus Creator/9  "1_L_x"
  Rate Transition1/1 -> Bus Creator/10  "1_L_y"

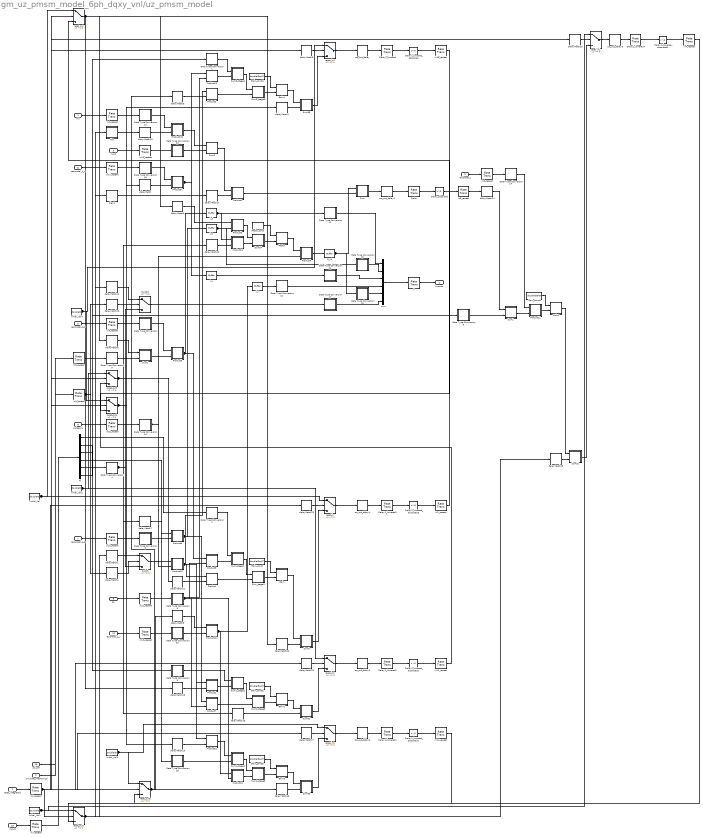
== system gm_uz_pmsm_model_6ph_dqxy_vnl/uz_pmsm_model ==
  reset_integrators : Inport  OutDataTypeStr=boolean  PortDimensions=1  SampleTime=5e-07
  simulate_mechanical : Inport  Port=2  OutDataTypeStr=boolean  PortDimensions=1  SampleTime=5e-07
  reciprocal_J : Inport  Port=3  OutDataTypeStr=single  PortDimensions=1  SampleTime=5e-07
  mu : Inport  Port=4  OutDataTypeStr=single  PortDimensions=1  SampleTime=5e-07
  M_n0 : Inport  Port=5  OutDataTypeStr=single  PortDimensions=1  SampleTime=5e-07
  reciprocal_L_d : Inport  Port=6  OutDataTypeStr=single  PortDimensions=1  SampleTime=5e-07
  reciprocal_L_q : Inport  Port=7  OutDataTypeStr=single  PortDimensions=1  SampleTime=5e-07
  R1 : Inport  Port=8  OutDataTypeStr=single  PortDimensions=1  SampleTime=5e-07
  polepairs : Inport  Port=9  OutDataTypeStr=single  PortDimensions=1  SampleTime=5e-07
  psi_pm : Inport  Port=10  OutDataTypeStr=single  PortDimensions=1  SampleTime=5e-07
  reciprocal_L_x : Inport  Port=11  OutDataTypeStr=single  PortDimensions=1  SampleTime=5e-07
  reciprocal_L_y : Inport  Port=12  OutDataTypeStr=single  PortDimensions=1  SampleTime=5e-07
  inputs : Inport  Port=13  OutDataTypeStr=single  PortDimensions=[6]  SampleTime=5e-07
  Abs : Subsystem
      mask Display: disp('NFP\nabs');
  Data Type Conversion1 : Subsystem
      mask Display: disp('NFP\nconv');
  Data Type Conversion10 : Subsystem
      mask Display: disp('NFP\nconv');
  Data Type Conversion11 : Subsystem
      mask Display: disp('NFP\nconv');
  Data Type Conversion12 : Subsystem
      mask Display: disp('NFP\nconv');
  Data Type Conversion13 : Subsystem
      mask Display: disp('NFP\nconv');
  Data Type Conversion14 : Subsystem
      mask Display: disp('NFP\nconv');
  Data Type Conversion15 : Subsystem
      mask Display: disp('NFP\nconv');
  Data Type Conversion16 : Subsystem
      mask Display: disp('NFP\nconv');
  Data Type Conversion17 : Subsystem
      mask Display: disp('NFP\nconv');
  Data Type Conversion18 : Subsystem
      mask Display: disp('NFP\nconv');
  Data Type Conversion19 : Subsystem
      mask Display: disp('NFP\nconv');
  Data Type Conversion2 : Subsystem
      mask Display: disp('NFP\nconv');
  Data Type Conversion20 : Subsystem
      mask Display: disp('NFP\nconv');
  Data Type Conversion21 : Subsystem
      mask Display: disp('NFP\nconv');
  Data Type Conversion22 : Subsystem
      mask Display: disp('NFP\nconv');
  Data Type Conversion3 : Subsystem
      mask Display: disp('NFP\nconv');
  Data Type Conversion4 : Subsystem
      mask Display: disp('NFP\nconv');
  Data Type Conversion5 : Subsystem
      mask Display: disp('NFP\nconv');
  Data Type Conversion6 : Subsystem
      mask Display: disp('NFP\nconv');
  Data Type Conversion7 : Subsystem
      mask Display: disp('NFP\nconv');
  Data Type Conversion8 : Subsystem
      mask Display: disp('NFP\nconv');
  Data Type Conversion9 : Subsystem
      mask Display: disp('NFP\nconv');
  Delay : RateTransition  InitialCondition=double(0)  OutPortSampleTimeOpt=Multiple of input port sample time  OutPortSampleTimeMultiple=50
  Delay1_lowered{,1..4} (5 alike) : RateTransition  InitialCondition=double(0)  OutPortSampleTimeOpt=Multiple of input port sample time  OutPortSampleTimeMultiple=50
  Delay1_lowered_absorbed{,1..4} (5 alike) : Delay  DelayLength=0
  Delay_absorbed : Delay  DelayLength=0
  Factor : Subsystem
      mask Display: disp('NFP\nmul');
  Factor_const : Constant  Value=double(1.5)  OutDataTypeStr=double  SampleTime=1e-08
  Gain : Subsystem
      mask Display: disp('NFP\nmul');
  Gain1 : Subsystem
      mask Display: disp('NFP\nmul');
  Gain2 : Subsystem
      mask Display: disp('NFP\nmul');
  Gain3 : Subsystem
      mask Display: disp('NFP\nmul');
  Gain4 : Subsystem
      mask Display: disp('NFP\nmul');
  Gain_const{,1..4} (5 alike) : Constant  Value=double(5e-07)  OutDataTypeStr=double  SampleTime=1e-08
  I_x : hdlmdlgenlib/Buffer
  I_y : hdlmdlgenlib/Buffer
  Initial_Val{,1..4} (5 alike) : Constant  Value=double(0)  OutDataTypeStr=double  SampleTime=1e-08
  M_Mi : hdlmdlgenlib/Buffer
  Product : Subsystem
      mask Display: disp('NFP\nmul');
  Product1 : Subsystem
      mask Display: disp('NFP\nmul');
  Product10 : Subsystem
      mask Display: disp('NFP\nmul');
  Product11 : Subsystem
      mask Display: disp('NFP\nmul');
  Product111 : Subsystem
      mask Display: disp('NFP\nmul');
  Product12 : Subsystem
      mask Display: disp('NFP\nmul');
  Product121 : Subsystem
      mask Display: disp('NFP\nmul');
  Product13 : Subsystem
      mask Display: disp('NFP\nmul');
  Product2 : Subsystem
      mask Display: disp('NFP\nmul');
  Product21 : Subsystem
      mask Display: disp('NFP\nmul');
  Product3 : Subsystem
      mask Display: disp('NFP\nmul');
  Product31 : Subsystem
      mask Display: disp('NFP\nmul');
  Product4 : Subsystem
      mask Display: disp('NFP\nmul');
  Product5 : Subsystem
      mask Display: disp('NFP\nmul');
  Product6 : Subsystem
      mask Display: disp('NFP\nmul');
  Product7 : Subsystem
      mask Display: disp('NFP\nmul');
  Product8 : Subsystem
      mask Display: disp('NFP\nmul');
  Product9 : Subsystem
      mask Display: disp('NFP\nmul');
  Product91 : Subsystem
      mask Display: disp('NFP\nmul');
  Sign1 : Subsystem
      mask Display: disp('NFP\nsignum');
  Sum : Subsystem
      mask Display: disp('NFP\nadd');
  Sum1 : Subsystem
      mask Display: disp('NFP\nadd');
  Sum1_stage2 : Subsystem
      mask Display: disp('NFP\nadd');
  Sum1_stage3 : Subsystem
      mask Display: disp('NFP\nadd');
  Sum2 : Subsystem
      mask Display: disp('NFP\nadd');
  Sum3 : Subsystem
      mask Display: disp('NFP\nadd');
  Sum31 : Subsystem
      mask Display: disp('NFP\nadd');
  Sum32 : Subsystem
      mask Display: disp('NFP\nadd');
  Sum33 : Subsystem
      mask Display: disp('NFP\nadd');
  Sum34 : Subsystem
      mask Display: disp('NFP\nadd');
  Sum35 : Subsystem
      mask Display: disp('NFP\nadd');
  Sum3_stage2 : Subsystem
      mask Display: disp('NFP\nadd');
  Sum3_stage3 : Subsystem
      mask Display: disp('NFP\nadd');
  Sum4_stage2 : Subsystem
      mask Display: disp('NFP\nadd');
  Sum4_stage3 : Subsystem
      mask Display: disp('NFP\nadd');
  Sum5 : Subsystem
      mask Display: disp('NFP\nadd');
  Sum_stage2 : Subsystem
      mask Display: disp('NFP\nadd');
  Sum_stage3 : Subsystem
      mask Display: disp('NFP\nadd');
  Switch : Switch  Criteria=u2 ~= 0  Threshold=double(0)  OutDataTypeStr=double  SampleTime=1e-08  SaturateOnIntegerOverflow=off  InputSameDT=off
  Switch1 : Switch  Criteria=u2 ~= 0  Threshold=double(0)  OutDataTypeStr=double  SampleTime=1e-08  SaturateOnIntegerOverflow=off  InputSameDT=off
  crp_out_delay{,1..5} (6 alike) : Delay  DelayLength=double(1)  InitialCondition=0  SampleTime=1e-08
  delayMatch{,1..26} (27 alike) : Delay  DelayLength=double(1)  InitialCondition=0  SampleTime=1e-08
  i_d : hdlmdlgenlib/Buffer
  i_q : hdlmdlgenlib/Buffer
  in0_repeat : RateTransition  Integrity=off  Deterministic=off  OutPortSampleTimeOpt=Multiple of input port sample time  OutPortSampleTimeMultiple=1/50
  in10_repeat : RateTransition  Integrity=off  Deterministic=off  OutPortSampleTimeOpt=Multiple of input port sample time  OutPortSampleTimeMultiple=1/50
  in11_repeat : RateTransition  Integrity=off  Deterministic=off  OutPortSampleTimeOpt=Multiple of input port sample time  OutPortSampleTimeMultiple=1/50
  in12_repeat : RateTransition  Integrity=off  Deterministic=off  OutPortSampleTimeOpt=Multiple of input port sample time  OutPortSampleTimeMultiple=1/50
  in13_repeat : RateTransition  Integrity=off  Deterministic=off  OutPortSampleTimeOpt=Multiple of input port sample time  OutPortSampleTimeMultiple=1/50
  in14_repeat : RateTransition  Integrity=off  Deterministic=off  OutPortSampleTimeOpt=Multiple of input port sample time  OutPortSampleTimeMultiple=1/50
  in15_repeat : RateTransition  Integrity=off  Deterministic=off  OutPortSampleTimeOpt=Multiple of input port sample time  OutPortSampleTimeMultiple=1/50
  in16_repeat : RateTransition  Integrity=off  Deterministic=off  OutPortSampleTimeOpt=Multiple of input port sample time  OutPortSampleTimeMultiple=1/50
  in17_repeat : RateTransition  Integrity=off  Deterministic=off  OutPortSampleTimeOpt=Multiple of input port sample time  OutPortSampleTimeMultiple=1/50
  in18_repeat : RateTransition  Integrity=off  Deterministic=off  OutPortSampleTimeOpt=Multiple of input port sample time  OutPortSampleTimeMultiple=1/50
  in1_repeat : RateTransition  Integrity=off  Deterministic=off  OutPortSampleTimeOpt=Multiple of input port sample time  OutPortSampleTimeMultiple=1/50
  in2_repeat : RateTransition  Integrity=off  Deterministic=off  OutPortSampleTimeOpt=Multiple of input port sample time  OutPortSampleTimeMultiple=1/50
  in3_repeat : RateTransition  Integrity=off  Deterministic=off  OutPortSampleTimeOpt=Multiple of input port sample time  OutPortSampleTimeMultiple=1/50
  in4_repeat : RateTransition  Integrity=off  Deterministic=off  OutPortSampleTimeOpt=Multiple of input port sample time  OutPortSampleTimeMultiple=1/50
  in5_repeat : RateTransition  Integrity=off  Deterministic=off  OutPortSampleTimeOpt=Multiple of input port sample time  OutPortSampleTimeMultiple=1/50
  in6_repeat : RateTransition  Integrity=off  Deterministic=off  OutPortSampleTimeOpt=Multiple of input port sample time  OutPortSampleTimeMultiple=1/50
  in7_repeat : RateTransition  Integrity=off  Deterministic=off  OutPortSampleTimeOpt=Multiple of input port sample time  OutPortSampleTimeMultiple=1/50
  in8_repeat : RateTransition  Integrity=off  Deterministic=off  OutPortSampleTimeOpt=Multiple of input port sample time  OutPortSampleTimeMultiple=1/50
  in9_repeat : RateTransition  Integrity=off  Deterministic=off  OutPortSampleTimeOpt=Multiple of input port sample time  OutPortSampleTimeMultiple=1/50
  mux : Mux  Inputs=6
  reset_in{,1..4} (5 alike) : Switch  Criteria=u2 ~= 0  Threshold=double(0)  OutDataTypeStr=double  SampleTime=1e-08  SaturateOnIntegerOverflow=off  InputSameDT=off
  reset_out{,1..4} (5 alike) : Switch  Criteria=u2 ~= 0  Threshold=double(0)  OutDataTypeStr=double  SampleTime=1e-08  SaturateOnIntegerOverflow=off  InputSameDT=off
  t : RateTransition  InitialCondition=double(0)  OutPortSampleTimeOpt=Multiple of input port sample time  OutPortSampleTimeMultiple=50
  t1 : Demux  Outputs=6
  outputs : Outport  SampleTime=5e-07
  wires:
  in14_repeat/1 -> reset_out3/3
  in11_repeat/1 -> reset_out2/3
  in4_repeat/1 -> reset_out1/3
  Data Type Conversion5/1(Out1) -> Sum1/2(In2)
  Data Type Conversion21/1(Out1) -> mux/3
  Data Type Conversion17/1(Out1) -> mux/6
  Product7/1(Out1) -> Sum1_stage3/2(In2)
  Product4/1(Out1) -> Sum/2(In2)
  Data Type Conversion3/1(Out1) -> Sum1_stage2/1(In1)
  t1/2 -> Data Type Conversion3/1(In1)
  Product2/1(Out1) -> Sum3_stage3/2(In2)
  in2_repeat/1 -> reset_out/3
  Data Type Conversion18/1(Out1) -> Sum4_stage2/2(In2)
  Product/1(Out1) -> Sum_stage3/2(In2)
  t1/1 -> Data Type Conversion2/1(In1)
  Data Type Conversion11/1(Out1) -> mux/1
  Product6/1(Out1) -> i_q/1, Product7/1(In1)
  Initial_Val2/1 -> reset_out2/1, reset_in2/1
  Product111/1(Out1) -> Product12/1(In1), I_y/1
  Initial_Val3/1 -> reset_out3/1, reset_in3/1
  Initial_Val4/1 -> reset_out4/1, reset_in4/1
  Data Type Conversion10/1(Out1) -> Product10/2(In2), Product9/2(In2)
  t1/3 -> Data Type Conversion1/1(In1)
  i_d/1 -> Product21/1(In1), Data Type Conversion11/1(In1)
  Data Type Conversion6/1(Out1) -> Product7/2(In2), Product8/2(In2), Product13/2(In2), Product12/2(In2)
  reset_integrators/1 -> in1_repeat/1
  simulate_mechanical/1 -> in3_repeat/1
  M_n0/1 -> in16_repeat/1
  reciprocal_L_d/1 -> in8_repeat/1
  reciprocal_L_q/1 -> in10_repeat/1
  psi_pm/1 -> in9_repeat/1
  reciprocal_L_x/1 -> in17_repeat/1
  inputs/1 -> in7_repeat/1
  t/1 -> outputs/1
  crp_out_delay1/1 -> Delay/1
  crp_out_delay3/1 -> Delay1_lowered2/1
  crp_out_delay5/1 -> Delay1_lowered4/1
  Delay/1 -> Delay_absorbed/1
  Delay1_lowered1/1 -> Delay1_lowered_absorbed1/1
  Initial_Val1/1 -> reset_out1/1, reset_in1/1
  Delay1_lowered2/1 -> Delay1_lowered_absorbed2/1
  Delay1_lowered_absorbed3/1 -> in2_repeat/1
  Delay1_lowered_absorbed4/1 -> in4_repeat/1
  crp_out_delay/1 -> Delay1_lowered/1
  in0_repeat/1 -> Data Type Conversion12/1(In1)
  in5_repeat/1 -> Data Type Conversion14/1(In1)
  in7_repeat/1 -> t1/1
  in8_repeat/1 -> Data Type Conversion7/1(In1)
  in9_repeat/1 -> Data Type Conversion9/1(In1)
  M_Mi/1 -> Sum/1(In1), Data Type Conversion16/1(In1)
  in12_repeat/1 -> Data Type Conversion6/1(In1)
  in13_repeat/1 -> Data Type Conversion20/1(In1)
  in15_repeat/1 -> Data Type Conversion10/1(In1)
  in16_repeat/1 -> Data Type Conversion13/1(In1)
  in6_repeat/1 -> delayMatch24/1
  Delay1_lowered_absorbed/1 -> in18_repeat/1
  Data Type Conversion4/1(Out1) -> Switch1/3, Switch/3
  reciprocal_L_y/1 -> in13_repeat/1
  Data Type Conversion15/1(Out1) -> mux/2
  delayMatch22/1 -> Sum3/2(In2)
  reset_in/1 -> crp_out_delay4/1
  reset_in1/1 -> crp_out_delay5/1
  in3_repeat/1 -> delayMatch2/1, delayMatch12/1
  Delay1_lowered/1 -> Delay1_lowered_absorbed/1
  Data Type Conversion2/1(Out1) -> Sum_stage2/1(In1)
  mu/1 -> in0_repeat/1
  delayMatch6/1 -> Sum2/1(In1)
  delayMatch7/1 -> Product6/1(In1)
  reset_in2/1 -> crp_out_delay3/1
  delayMatch3/1 -> Product2/2(In2)
  Initial_Val/1 -> reset_in/1, reset_out/1
  R1/1 -> in12_repeat/1
  crp_out_delay2/1 -> Delay1_lowered1/1
  Switch/1 -> Product10/1(In1)
  reciprocal_J/1 -> in5_repeat/1
  reset_in3/1 -> crp_out_delay2/1
  reset_out2/1 -> delayMatch19/1, delayMatch7/1, delayMatch21/1, delayMatch10/1
  Product10/1(Out1) -> Product/1(In1), Product2/1(In1), Product31/1(In1), Product1/1(In1)
  delayMatch14/1 -> Product4/2(In2)
  delayMatch9/1 -> Product3/1(In1)
  delayMatch13/1 -> Product121/2(In2)
  Product9/1(Out1) -> M_Mi/1
  Factor/1(Out1) -> Product9/1(In1)
  t1/5 -> Data Type Conversion4/1(In1)
  I_x/1 -> Data Type Conversion21/1(In1)
  Delay1_lowered_absorbed1/1 -> in14_repeat/1
  delayMatch4/1 -> Sum35/2(In2)
  reset_in4/1 -> crp_out_delay/1
  delayMatch19/1 -> Sum32/2(In2)
  Data Type Conversion1/1(Out1) -> Sum3_stage2/1(In1)
  delayMatch5/1 -> reset_in4/2
  delayMatch2/1 -> Switch/2
  Gain_const/1 -> Gain/1(In1)
  Product5/1(Out1) -> i_d/1, Product8/1(In1)
  Gain_const2/1 -> Gain2/1(In1)
  Sum1/1(Out1) -> Product11/2(In2)
  crp_out_delay4/1 -> Delay1_lowered3/1
  Delay1_lowered3/1 -> Delay1_lowered_absorbed3/1
  Gain_const4/1 -> Gain4/1(In1)
  Delay1_lowered_absorbed2/1 -> in11_repeat/1
  Data Type Conversion22/1(Out1) -> mux/4
  Sum_stage2/1(Out1) -> Sum_stage3/1(In1)
  Product13/1(Out1) -> Sum3_stage2/2(In2)
  delayMatch1/1 -> Switch/1
  Product11/1(Out1) -> Gain1/2(In2)
  Data Type Conversion7/1(Out1) -> Product5/1(In1)
  Sum1_stage3/1(Out1) -> Gain2/2(In2)
  Gain_const3/1 -> Gain3/1(In1)
  reset_out3/1 -> delayMatch16/1, delayMatch3/1, delayMatch8/1
  Sum33/1(Out1) -> reset_in3/3
  Sum2/1(Out1) -> Product5/2(In2)
  Data Type Conversion9/1(Out1) -> Sum2/2(In2)
  Sum4_stage2/1(Out1) -> Sum4_stage3/1(In1)
  mux/1 -> t/1
  Sum4_stage3/1(Out1) -> Gain3/2(In2)
  Data Type Conversion14/1(Out1) -> Product11/1(In1)
  Sum3/1(Out1) -> reset_in/3
  delayMatch16/1 -> Sum33/2(In2)
  polepairs/1 -> in15_repeat/1
  Abs/1(Out1) -> delayMatch13/1
  in10_repeat/1 -> Data Type Conversion8/1(In1)
  Sum32/1(Out1) -> reset_in2/3
  Data Type Conversion13/1(Out1) -> Sum5/2(In2)
  reset_out/1 -> delayMatch22/1, delayMatch6/1, delayMatch9/1, delayMatch18/1
  Sum35/1(Out1) -> reset_in4/3
  Switch1/1 -> Data Type Conversion17/1(In1)
  Sum3_stage3/1(Out1) -> Gain4/2(In2)
  Product12/1(Out1) -> Sum4_stage3/2(In2)
  Gain1/1(Out1) -> Sum31/1(In1)
  delayMatch10/1 -> Product21/2(In2)
  Sum34/1(Out1) -> Factor/2(In2)
  Product8/1(Out1) -> Sum_stage2/2(In2)
  reset_out1/1 -> delayMatch11/1, delayMatch1/1, Sign1/1(In1), Abs/1(In1), delayMatch25/1
  Gain3/1(Out1) -> Sum33/1(In1)
  Sum5/1(Out1) -> Product4/1(In1)
  delayMatch24/1 -> Sum1/1(In1)
  Product3/1(Out1) -> Sum34/1(In1)
  Data Type Conversion19/1(Out1) -> Product91/1(In1)
  Product21/1(Out1) -> Sum34/2(In2)
  I_y/1 -> Data Type Conversion22/1(In1)
  Sum_stage3/1(Out1) -> Gain/2(In2)
  Delay1_lowered4/1 -> Delay1_lowered_absorbed4/1
  Factor_const/1 -> Factor/1(In1)
  delayMatch15/1 -> Product31/2(In2)
  Gain_const1/1 -> Gain1/1(In1)
  delayMatch11/1 -> Switch1/1
  delayMatch17/1 -> reset_in3/2
  Data Type Conversion20/1(Out1) -> Product111/2(In2)
  Gain2/1(Out1) -> Sum32/1(In1)
  Product91/1(Out1) -> Product13/1(In1), I_x/1
  delayMatch12/1 -> Switch1/2
  t1/6 -> Data Type Conversion5/1(In1)
  delayMatch25/1 -> Sum31/2(In2)
  Product1/1(Out1) -> Sum1_stage2/2(In2)
  Sum31/1(Out1) -> reset_in1/3
  in17_repeat/1 -> Data Type Conversion19/1(In1)
  Delay_absorbed/1 -> in6_repeat/1
  Gain4/1(Out1) -> Sum35/1(In1)
  reset_out4/1 -> delayMatch/1, delayMatch4/1, delayMatch15/1
  Data Type Conversion8/1(Out1) -> Product6/2(In2)
  delayMatch21/1 -> Product/2(In2)
  t1/4 -> Data Type Conversion18/1(In1)
  Gain/1(Out1) -> Sum3/1(In1)
  Sign1/1(Out1) -> delayMatch14/1
  Data Type Conversion12/1(Out1) -> Product121/1(In1)
  Product121/1(Out1) -> Sum5/1(In1)
  delayMatch18/1 -> Product1/2(In2)
  delayMatch8/1 -> Product111/1(In1)
  Data Type Conversion16/1(Out1) -> mux/5
  delayMatch20/1 -> reset_in2/2
  in1_repeat/1 -> reset_out1/2, delayMatch20/1, reset_out/2, reset_out2/2, delayMatch26/1, reset_out3/2, reset_out4/2, delayMatch17/1, delayMatch5/1, delayMatch23/1
  delayMatch/1 -> Product91/2(In2)
  delayMatch23/1 -> reset_in/2
  Sum1_stage2/1(Out1) -> Sum1_stage3/1(In1)
  in18_repeat/1 -> reset_out4/3
  Sum3_stage2/1(Out1) -> Sum3_stage3/1(In1)
  delayMatch26/1 -> reset_in1/2
  Product31/1(Out1) -> Sum4_stage2/1(In1)
  Sum/1(Out1) -> crp_out_delay1/1
  i_q/1 -> Data Type Conversion15/1(In1), Product3/2(In2)
